simulink model "SnakeRobotPDMatlab"  (R2015b)
settings: Solver=FixedStepAuto  StartTime=0  StopTime=tmax  FixedStep=tpaso  RelTol=1e-3
values from neighbouring files (symbols this model uses):
  Bm = 1.34e-4    (= 0.000134)    [PreSim.m]
  c1 = 0.45    [PreSim.m]
  c2 = 3    [PreSim.m]
  c3 = 0.5    [PreSim.m]
  c4 = 20    [PreSim.m]
  Jm = 3.2e-6    (= 3.2e-06)    [PreSim.m]
  Ko = 0.036    [PreSim.m]
  Lm = 2e-3    (= 0.002)    [PreSim.m]
  Ms = 1    [PreSim.m]
  N = 3    [PreSim.m]
  Rm = 10.9    [PreSim.m]
  tmax = 50    [GeneticPrinterMotor_2_Redefinition.m]    (also in GeneticPrinterMotor_3_SelectionCrossoverAdjust.m; GeneticPrinterMotor_4_MicroGA.m; PreSim.m = 100)
  tpaso = 0.01    [GeneticPrinterMotor.m]    (also in GeneticPrinterMotor_2_Redefinition.m; GeneticPrinterMotor_3_SelectionCrossoverAdjust.m; GeneticPrinterMotor_4_MicroGA.m; GeneticSnakeP.m)
settings Model: Creator=Christian Dos Santos  LastModifiedBy=Christian Dos Santos

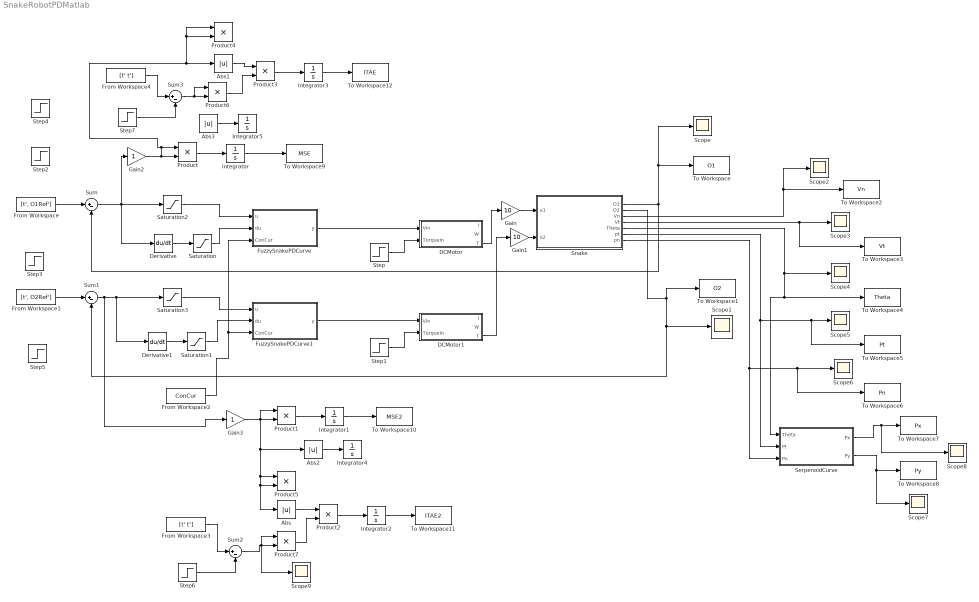
== system SnakeRobotPDMatlab ==
  Abs{,1..3} (4 alike) : Abs
  DCMotor : Subsystem
  DCMotor1 : Subsystem
  Derivative : Derivative
  Derivative1 : Derivative
  From Workspace : FromWorkspace  VariableName=[t', O1Ref']  SampleTime=tpaso
  From Workspace1 : FromWorkspace  VariableName=[t', O2Ref']  SampleTime=tpaso
  From Workspace2 : FromWorkspace  VariableName=ConCur  SampleTime=tpaso
  From Workspace3 : FromWorkspace  VariableName=[t' t']  SampleTime=tpaso
  From Workspace4 : FromWorkspace  VariableName=[t' t']  SampleTime=tpaso
  FuzzySnakePDCurve : MATLAB Function  TreatAsAtomicUnit=on
  FuzzySnakePDCurve1 : MATLAB Function  TreatAsAtomicUnit=on
  Gain : Gain  Gain=10
  Gain1 : Gain  Gain=10
  Gain2 : Gain
  Gain3 : Gain
  Integrator{,1..5} (6 alike) : Integrator
  Product{,1..7} (8 alike) : Product
  Saturation{,1..3} (4 alike) : Saturate  UpperLimit=0.1  LowerLimit=-0.1
  Scope{,1..9} (10 alike) : Scope
  SerpenoidCurve : Subsystem
  Snake : Subsystem
  Step : Step  Time=0  After=0.0018  SampleTime=tpaso
  Step1 : Step  Time=0  After=0.0008  SampleTime=tpaso
  Step2 : Step  Time=0  After=0.1  SampleTime=tpaso
  Step3 : Step  Time=0  After=0.1  SampleTime=tpaso
  Step4 : Step  Time=tmax/2  Before=0.1  After=-0.1  SampleTime=tpaso
  Step5 : Step  Time=tmax/2  Before=0.1  After=-0.1  SampleTime=tpaso
  Step6 : Step  Time=tmax/2  After=tmax/2  SampleTime=tpaso
  Step7 : Step  Time=tmax/2  After=tmax/2  SampleTime=tpaso
  Sum{,1..3} (4 alike) : Sum  Inputs=|+-
  To Workspace : ToWorkspace  VariableName=O1  SampleTime=-1
  To Workspace1 : ToWorkspace  VariableName=O2  SampleTime=-1
  To Workspace10 : ToWorkspace  VariableName=MSE2  SampleTime=-1
  To Workspace11 : ToWorkspace  VariableName=ITAE2  SampleTime=-1
  To Workspace12 : ToWorkspace  VariableName=ITAE  SampleTime=-1
  To Workspace2 : ToWorkspace  VariableName=Vn  SampleTime=-1
  To Workspace3 : ToWorkspace  VariableName=Vt  SampleTime=-1
  To Workspace4 : ToWorkspace  VariableName=Theta  SampleTime=-1
  To Workspace5 : ToWorkspace  VariableName=Pt  SampleTime=-1
  To Workspace6 : ToWorkspace  VariableName=Pn  SampleTime=-1
  To Workspace7 : ToWorkspace  VariableName=Px  SampleTime=-1
  To Workspace8 : ToWorkspace  VariableName=Py  SampleTime=-1
  To Workspace9 : ToWorkspace  VariableName=MSE  SampleTime=-1
  wires:
  FuzzySnakePDCurve/1(y) -> DCMotor/1(Vin)
  FuzzySnakePDCurve1/1(y) -> DCMotor1/1(Vin)
  Snake/2(O2) -> Scope1/1, Sum1/2, To Workspace1/1
  Step/1 -> DCMotor/2(TorqueIn)
  Step1/1 -> DCMotor1/2(TorqueIn)
  Snake/1(O1) -> Sum/2, Scope/1, To Workspace/1
  Snake/3(Vn) -> Scope2/1, To Workspace2/1
  Snake/4(Vt) -> To Workspace3/1, Scope3/1
  Snake/5(Theta) -> Scope4/1, SerpenoidCurve/1(Theta), To Workspace4/1
  Snake/6(pt) -> SerpenoidCurve/2(Pt), To Workspace5/1, Scope5/1
  Snake/7("pn ") -> SerpenoidCurve/3(Pn), To Workspace6/1, Scope6/1
  Gain/1 -> Snake/1(u1)
  DCMotor/3(T) -> Gain/1
  DCMotor1/3(T) -> Gain1/1
  Gain1/1 -> Snake/2(u2)
  Derivative/1 -> Saturation/1
  Saturation2/1 -> FuzzySnakePDCurve/1(u)
  Saturation1/1 -> FuzzySnakePDCurve1/2(du)
  Derivative1/1 -> Saturation1/1
  Saturation3/1 -> FuzzySnakePDCurve1/1(u)
  SerpenoidCurve/1(Px) -> Scope8/1, To Workspace7/1
  SerpenoidCurve/2(Py) -> Scope7/1, To Workspace8/1
  Saturation/1 -> FuzzySnakePDCurve/2(du)
  Sum/1 -> Gain2/1, Derivative/1, Saturation2/1
  Product/1 -> Integrator/1
  Product3/1 -> Integrator3/1
  Integrator3/1 -> To Workspace12/1
  Gain2/1 -> Product/2, Product/1, Product4/1, Product4/2, Abs1/1
  Abs3/1 -> Integrator5/1
  Integrator/1 -> To Workspace9/1
  Sum1/1 -> Gain3/1, Derivative1/1, Saturation3/1
  Product1/1 -> Integrator1/1
  Gain3/1 -> Product5/1, Product5/2, Abs/1, Abs2/1, Product1/2, Product1/1
  Product2/1 -> Integrator2/1
  Integrator2/1 -> To Workspace11/1
  Abs2/1 -> Integrator4/1
  Integrator1/1 -> To Workspace10/1
  From Workspace2/1 -> FuzzySnakePDCurve1/3(ConCur), FuzzySnakePDCurve/3(ConCur)
  Product6/1 -> Product3/2
  Abs1/1 -> Product3/1
  Product7/1 -> Product2/2
  Abs/1 -> Product2/1
  From Workspace3/1 -> Sum2/1
  Step6/1 -> Sum2/2
  Sum2/1 -> Scope9/1, Product7/1, Product7/2
  Step7/1 -> Sum3/2
  From Workspace4/1 -> Sum3/1
  Sum3/1 -> Product6/1, Product6/2
  From Workspace/1 -> Sum/1
  From Workspace1/1 -> Sum1/1

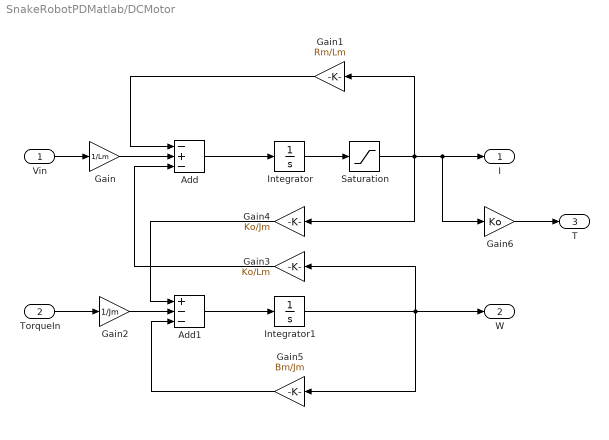
== system SnakeRobotPDMatlab/DCMotor ==
  Vin : Inport
  TorqueIn : Inport  Port=2
  Add : Sum  Inputs=-+-
  Add1 : Sum  Inputs=+--
  Gain : Gain  Gain=1/Lm
  Gain1 : Gain  Gain=Rm/Lm
  Gain2 : Gain  Gain=1/Jm
  Gain3 : Gain  Gain=Ko/Lm
  Gain4 : Gain  Gain=Ko/Jm
  Gain5 : Gain  Gain=Bm/Jm
  Gain6 : Gain  Gain=Ko
  Integrator : Integrator
  Integrator1 : Integrator
  Saturation : Saturate  UpperLimit=3.5  LowerLimit=-3.5
  I : Outport
  W : Outport  Port=2
  T : Outport  Port=3
  wires:
  Vin/1 -> Gain/1
  Gain/1 -> Add/2
  Add/1 -> Integrator/1
  Integrator/1 -> Saturation/1
  Saturation/1 -> Gain4/1, Gain1/1, Gain6/1, I/1
  Gain1/1 -> Add/1
  TorqueIn/1 -> Gain2/1
  Gain2/1 -> Add1/2
  Add1/1 -> Integrator1/1
  Integrator1/1 -> Gain5/1, Gain3/1, W/1
  Gain3/1 -> Add/3
  Gain4/1 -> Add1/1
  Gain5/1 -> Add1/3
  Gain6/1 -> T/1

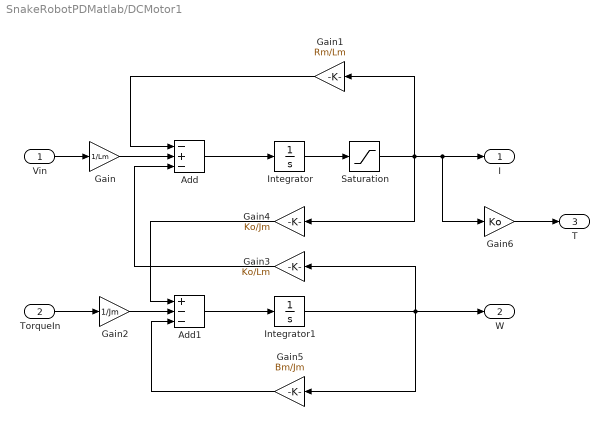
== system SnakeRobotPDMatlab/DCMotor1 ==
  Vin : Inport
  TorqueIn : Inport  Port=2
  Add : Sum  Inputs=-+-
  Add1 : Sum  Inputs=+--
  Gain : Gain  Gain=1/Lm
  Gain1 : Gain  Gain=Rm/Lm
  Gain2 : Gain  Gain=1/Jm
  Gain3 : Gain  Gain=Ko/Lm
  Gain4 : Gain  Gain=Ko/Jm
  Gain5 : Gain  Gain=Bm/Jm
  Gain6 : Gain  Gain=Ko
  Integrator : Integrator
  Integrator1 : Integrator
  Saturation : Saturate  UpperLimit=3.5  LowerLimit=-3.5
  I : Outport
  W : Outport  Port=2
  T : Outport  Port=3
  wires:
  Vin/1 -> Gain/1
  Gain/1 -> Add/2
  Add/1 -> Integrator/1
  Integrator/1 -> Saturation/1
  Saturation/1 -> Gain4/1, Gain1/1, Gain6/1, I/1
  Gain1/1 -> Add/1
  TorqueIn/1 -> Gain2/1
  Gain2/1 -> Add1/2
  Add1/1 -> Integrator1/1
  Integrator1/1 -> Gain5/1, Gain3/1, W/1
  Gain3/1 -> Add/3
  Gain4/1 -> Add1/1
  Gain5/1 -> Add1/3
  Gain6/1 -> T/1

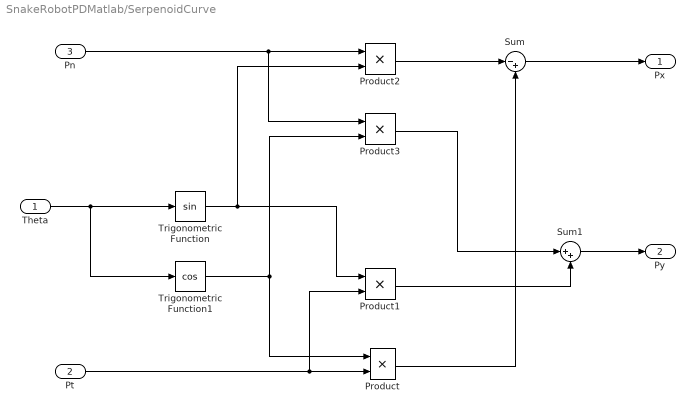
== system SnakeRobotPDMatlab/SerpenoidCurve ==
  Theta : Inport
  Pt : Inport  Port=2
  Pn : Inport  Port=3
  Product{,1..3} (4 alike) : Product
  Sum : Sum  Inputs=|-+
  Sum1 : Sum  Inputs=|++
  Trigonometric Function : Trigonometry
  Trigonometric Function1 : Trigonometry  Operator=cos
  Px : Outport
  Py : Outport  Port=2
  wires:
  Theta/1 -> Trigonometric Function1/1, Trigonometric Function/1
  Pn/1 -> Product3/1, Product2/1
  Trigonometric Function/1 -> Product2/2, Product1/1
  Trigonometric Function1/1 -> Product/1, Product3/2
  Pt/1 -> Product1/2, Product/2
  Product2/1 -> Sum/1
  Product/1 -> Sum/2
  Product1/1 -> Sum1/2
  Product3/1 -> Sum1/1
  Sum1/1 -> Py/1
  Sum/1 -> Px/1

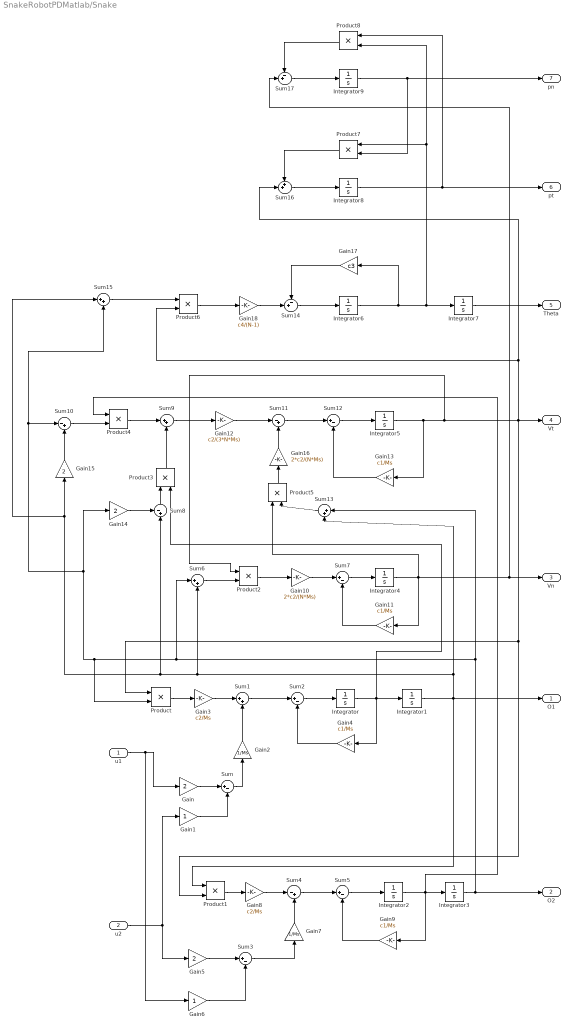
== system SnakeRobotPDMatlab/Snake ==
  u1 : Inport
  u2 : Inport  Port=2
  Gain{,5,14..15} (4 alike) : Gain  Gain=2
  Gain1 : Gain
  Gain10 : Gain  Gain=2*c2/(N*Ms)
  Gain{4,9,11,13} (4 alike) : Gain  Gain=c1/Ms
  Gain12 : Gain  Gain=c2/(3*N*Ms)
  Gain16 : Gain  Gain=2*c2/(N*Ms)
  Gain17 : Gain  Gain=c3
  Gain18 : Gain  Gain=c4/(N-1)
  Gain2 : Gain  Gain=1/Ms
  Gain3 : Gain  Gain=c2/Ms
  Gain6 : Gain
  Gain7 : Gain  Gain=1/Ms
  Gain8 : Gain  Gain=c2/Ms
  Integrator{,1..9} (10 alike) : Integrator
  Product{,1..8} (9 alike) : Product
  Sum{,2..3,5,7,12} (6 alike) : Sum  Inputs=|+-
  Sum{1,6,9,13,15} (5 alike) : Sum  Inputs=|++
  Sum10 : Sum  Inputs=|-+
  Sum11 : Sum  Inputs=|-+
  Sum14 : Sum  Inputs=-+|
  Sum16 : Sum  Inputs=++|
  Sum17 : Sum  Inputs=-+|
  Sum4 : Sum  Inputs=|-+
  Sum8 : Sum  Inputs=-+|
  O1 : Outport
  O2 : Outport  Port=2
  Vn : Outport  Port=3
  Vt : Outport  Port=4
  Theta : Outport  Port=5
  pt : Outport  Port=6
  "pn " : Outport  Port=7
  wires:
  u1/1 -> Gain6/1, Gain/1
  Gain/1 -> Sum/1
  u2/1 -> Gain1/1, Gain5/1
  Gain1/1 -> Sum/2
  Sum/1 -> Gain2/1
  Product/1 -> Gain3/1
  Sum1/1 -> Sum2/1
  Sum2/1 -> Integrator/1
  Integrator/1 -> Gain4/1, Product3/2, Integrator1/1
  Gain2/1 -> Sum1/2
  Gain3/1 -> Sum1/1
  Gain4/1 -> Sum2/2
  Gain5/1 -> Sum3/1
  Gain6/1 -> Sum3/2
  Sum3/1 -> Gain7/1
  Gain7/1 -> Sum4/2
  Gain8/1 -> Sum4/1
  Product1/1 -> Gain8/1
  Sum4/1 -> Sum5/1
  Sum5/1 -> Integrator2/1
  Integrator2/1 -> Gain9/1, Product4/1, Integrator3/1
  Gain9/1 -> Sum5/2
  Sum6/1 -> Product2/2
  Product2/1 -> Gain10/1
  Gain10/1 -> Sum7/1
  Sum7/1 -> Integrator4/1
  Integrator4/1 -> Vn/1, Sum17/2, Gain11/1, Product5/1
  Gain11/1 -> Sum7/2
  Sum8/1 -> Product3/1
  Product3/1 -> Sum9/2
  Product4/1 -> Sum9/1
  Sum10/1 -> Product4/2
  Sum9/1 -> Gain12/1
  Gain12/1 -> Sum11/1
  Sum11/1 -> Sum12/1
  Sum12/1 -> Integrator5/1
  Integrator5/1 -> Gain13/1, Product/1, Product1/2, Vt/1, Product6/2, Sum16/2, Product2/1
  Gain13/1 -> Sum12/2
  Gain14/1 -> Sum8/1
  Gain15/1 -> Sum10/2
  Integrator1/1 -> Product1/1, O1/1, Sum6/2, Sum8/2, Sum15/1, Gain15/1, Sum13/2
  Gain16/1 -> Sum11/2
  Product5/1 -> Gain16/1
  Sum13/1 -> Product5/2
  Integrator6/1 -> Product8/2, Product7/1, Integrator7/1, Gain17/1
  Gain17/1 -> Sum14/1
  Sum14/1 -> Integrator6/1
  Gain18/1 -> Sum14/2
  Product6/1 -> Gain18/1
  Sum15/1 -> Product6/1
  Integrator7/1 -> Theta/1
  Sum16/1 -> Integrator8/1
  Product7/1 -> Sum16/1
  Sum17/1 -> Integrator9/1
  Product8/1 -> Sum17/1
  Integrator9/1 -> "pn "/1, Product7/2
  Integrator8/1 -> Product8/1, pt/1
  Integrator3/1 -> Sum13/1, Sum6/1, Product/2, Sum15/2, Sum10/1, Gain14/1, O2/1

== matlab function SnakeRobotPDMatlab/FuzzySnakePDCurve1 ==
  data: u input; du input; y output; ConCur input
function y = fcn(u, du, ConCur)
%#codegen
pasou = 0.001;
pasodu = 0.001;
Maxpointu = 200;
Maxpointdu = 200;
% uAux = floor( (u + 0.1)/ pasou + 1 );
uAux = round( (u + 0.1)/ pasou + 1 );
% duAux = floor( (du + 0.1)/ pasodu + 1 );
duAux = round( (du + 0.1)/ pasodu + 1 );
CurveInd = duAux + (uAux - 1)*Maxpointdu;
if CurveInd >= Maxpointu*Maxpointdu + 401
    CurveInd = Maxpointu*Maxpointdu;
end
if CurveInd <= 0
   CurveInd = 1;
end
y = ConCur(CurveInd);

== matlab function SnakeRobotPDMatlab/FuzzySnakePDCurve ==
  data: u input; du input; y output; ConCur input
function y = fcn(u, du,ConCur)
%#codegen
pasou = 0.001;
pasodu = 0.001;
Maxpointu = 200;
Maxpointdu = 200;
% uAux = floor( (u + 0.1)/ pasou + 1 );
uAux = round( (u + 0.1)/ pasou + 1 );
% duAux = floor( (du + 0.1)/ pasodu + 1 );
duAux = round( (du + 0.1)/ pasodu + 1 );
CurveInd = duAux + (uAux - 1)*Maxpointdu;
if CurveInd >= Maxpointu*Maxpointdu + 401
    CurveInd = Maxpointu*Maxpointdu;
end
if CurveInd <= 0
   CurveInd = 1;
end
y = ConCur(CurveInd);
